simulink model "practicaControlTemperatura"  (R2025a)
settings: Solver=VariableStepAuto  StartTime=0.0  StopTime=1000  RelTol=1e-3
libraries: fuzblock x1
settings Model: Creator=Bremdow  LastModifiedBy=Bremdows

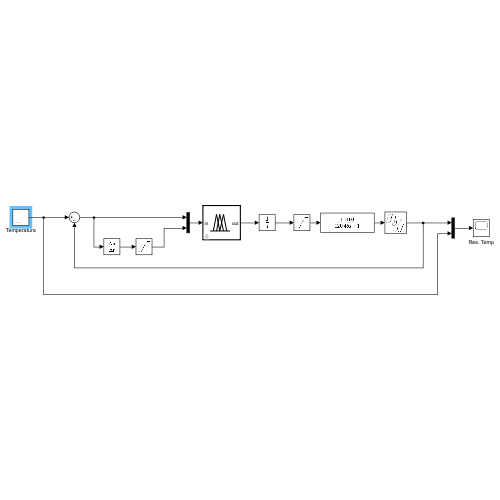
[thumbnail: Simulink's stored preview of the top-level diagram]
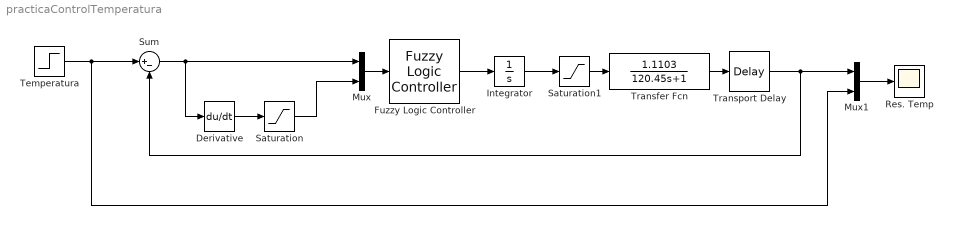
== system practicaControlTemperatura ==
  Derivative : Derivative
  Fuzzy Logic Controller : fuzblock/Fuzzy Logic  Controller  FIS='controlTemperatura.fis'  OutputSampleNumber=101  DataType=double  UseLookupTable=off  NumBreakpoints=10  FuzzifiedInputs=off  RuleFiringStrengths=off  RuleOutputs=off  AggregatedOutputs=off  SimulateUsing=Interpreted execution  OutOfRangeInputValueMessage=warning  NoRuleFiredMessage=warning  EmptyOutputFuzzySetMessage=warning
  Integrator : Integrator
  Mux : Mux  Inputs=2
  Mux1 : Mux  Inputs=2
  Res. Temp : Scope
      settings: ActiveDisplayYMinimum=-8.0582001167788935  ActiveDisplayYMaximum=72.523801051010054
  Saturation : Saturate  UpperLimit=4  LowerLimit=-4
  Saturation1 : Saturate  UpperLimit=100  LowerLimit=0
  Sum : Sum  Inputs=|+-
  Temperatura : Step  After=10  SampleTime=0
  Transfer Fcn : TransferFcn  Numerator=[1.1103]  Denominator=[120.45 1]
  Transport Delay : TransportDelay  DelayTime=12.78
  wires:
  Mux/1 -> Fuzzy Logic Controller/1
  Temperatura/1 -> Mux1/2, Sum/1
  Transfer Fcn/1 -> Transport Delay/1
  Mux1/1 -> Res. Temp/1
  Sum/1 -> Mux/1, Derivative/1
  Saturation/1 -> Mux/2
  Derivative/1 -> Saturation/1
  Fuzzy Logic Controller/1 -> Integrator/1
  Integrator/1 -> Saturation1/1
  Saturation1/1 -> Transfer Fcn/1
  Transport Delay/1 -> Mux1/1, Sum/2
